simulink model "invPendulumSim"  (Simulink 8.3)
settings: Solver=ode45  StartTime=0.0  StopTime=30  RelTol=1e-3
undefined symbols (not defined in the file or in its folder): invertedPendulum, invPendulumPlot, sigbuilder_block, wrap2Pi
settings Model: Creator=rbabuska  LastModifiedBy=yudhapane
settings OptimizationCC: ExpressionDepthLimit=2147483647
settings DebuggingCC: SolverPrmCheckMsg=none  FcnCallInpInsideContextMsg=EnableAllAsWarning

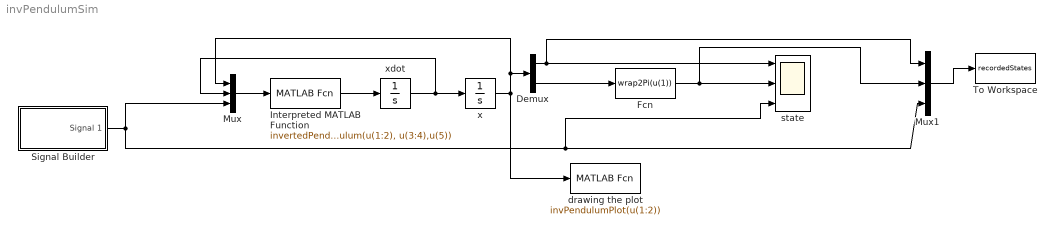
== system invPendulumSim ==
  Demux : Demux  Outputs=2
  Fcn : Fcn  Expr=wrap2Pi(u(1))
  Interpreted MATLAB Function : MATLABFcn  MATLABFcn=invertedPendulum(u(1:2), u(3:4),u(5))  OutputDimensions=2
  Mux : Mux  Inputs=3
  Mux1 : Mux  Inputs=3
  Signal Builder : Subsystem  Tag=STV Subsys  LoadFcn=sigbuilder_block('load',[634.966 5.58621 551.172 392.276 ]);  StartFcn=sigbuilder_block('start');  StopFcn=sigbuilder_block('stop');  ClipboardFcn=sigbuilder_block('clipboard');  mask(Sigbuilder block){}
      mask help: Simulink:masks:SigbuilderBlock_MD
      mask init:
      | if ~strcmp(get_param(bdroot(gcbh),'SimulationStatus'),'stopped') tuvar = sigbuilder_block('maskInit'); end
      settings: CopyFcn=sigbuilder_block('copy');  DeleteFcn=sigbuilder_block('delete');  ModelCloseFcn=sigbuilder_block('modelClose');  PreSaveFcn=sigbuilder_block('preSave');  PauseFcn=sigbuilder_block('pause')  ContinueFcn=sigbuilder_block('continue')  NameChangeFcn=sigbuilder_block('namechange');  OpenFcn=sigbuilder_block('open',[370.552 185.586 550.552 399.724 ]);  CloseFcn=sigbuilder_block('close');
      mask Display: plot(0, 0, 100, 100,[2, 2, 32, 32, 2], [68, 8, 8, 68, 68],[32, 2], [38, 38], [32, 19, 2],[53, 60, 44], [32, 17, 17, 2],[16, 16, 31, 31]);txt = getActiveGroup(gcbh);text(2, 100, txt,'verticalAlignment', 'top');
  To Workspace : ToWorkspace  VariableName=recordedStates  SaveFormat=Timeseries  SampleTime=-1
  drawing the plot : MATLABFcn  MATLABFcn=invPendulumPlot(u(1:2))  OutputDimensions=0
  state : Scope  NumInputPorts=3
      settings: YMin=-0.07~-0.05~-5  YMax=0~0.05~5
  x : Integrator  InitialCondition=[0, 0]
  xdot : Integrator  InitialCondition=[0, 0]
  wires:
  Interpreted MATLAB Function/1 -> xdot/1
  xdot/1 -> x/1, Mux/2
  Mux/1 -> Interpreted MATLAB Function/1
  x/1 -> Demux/1, Mux/1, drawing the plot/1
  Demux/2 -> Fcn/1
  Demux/1 -> Mux1/1, state/1
  Signal Builder/1(Signal 1) -> Mux1/3, state/3, Mux/3
  Mux1/1 -> To Workspace/1
  Fcn/1 -> Mux1/2, state/2

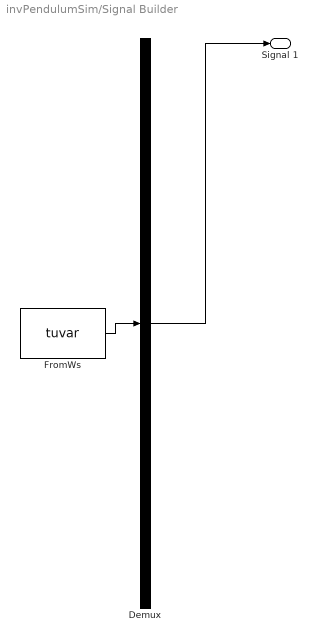
== system invPendulumSim/Signal Builder ==
  Demux : Demux  Tag=STV Demux  Outputs=1
  FromWs : FromWorkspace  Tag=STV FromWs  VariableName=tuvar  SampleTime=0  SigBuilderData=DataTag0  VnvData=DataTag1
      SigBuilderData=|
      | common.afterFinalStr = 'Extrapolate'
      | common.sampleTime = 0
      | dataSet.timeRange = [0 10]
      | dataSet.name = 'Group 1'
      | sbobj.Groups.Name = 'Group 1'
      | sbobj.Groups.Signals.Name = 'Signal 1'
      | sbobj.Groups.Signals.XData = [0 1 1 2 2 3 3 4 4 5 5 6 6 7 7 8 8 9 9 10]
      | sbobj.Groups.Signals.YData = [-0.1 -0.1 -5 -5 4.9 4.9 -5 -5 5 5 -5 -5 5 5 -5.1 -5.1 5 5 0 0]
  Signal 1 : Outport  Tag=STV Outport
  wires:
  Demux/1 -> Signal 1/1
  FromWs/1 -> Demux/1
